simulink model "sampleModel7293_pp_1_1_mu"  (R2018a)
settings: Solver=VariableStepAuto  StartTime=0.0  StopTime=10.0  RelTol=1e-3
undefined symbols (not defined in the file): DiscIntNeverNeededParam
libraries: simulink x367
(part 3 of 13)

== system sampleModel7293_pp_1_1_mu/cfblk181 ==
  cfblk1 : Inport
  Action Port : ActionPort  ActionType=else
  cfblk10 : Subsystem  TreatAsAtomicUnit=on
  cfblk3 : simulink/Continuous/PID Controller (2DOF)  Controller=PID  TimeDomain=Discrete-time  SampleTime=-1  IntegratorMethod=Forward Euler  FilterMethod=Forward Euler  Form=Parallel  UseFilter=on  ControllerParametersSource=internal  P=1  I=1  D=0  N=100  b=1  c=1  InitialConditionSource=internal  InitialConditionForIntegrator=0  InitialConditionForFilter=0  ExternalReset=none  LimitOutput=off  UpperSaturationLimit=inf  LowerSaturationLimit=-inf  LinearizeAsGain=off  AntiWindupMode=none  Kb=1  TrackingMode=off  Kt=1  PParamMin=[]  PParamMax=[]  IParamMin=[]  IParamMax=[]  DParamMin=[]  DParamMax=[]  NParamMin=[]  NParamMax=[]  bParamMin=[]  bParamMax=[]  cParamMin=[]  cParamMax=[]  KbParamMin=[]  KbParamMax=[]  KtParamMin=[]  KtParamMax=[]  POutMin=[]  POutMax=[]  IOutMin=[]  IOutMax=[]  DOutMin=[]  DOutMax=[]  NOutMin=[]  NOutMax=[]  bOutMin=[]  bOutMax=[]  cOutMin=[]  cOutMax=[]  KbOutMin=[]  KbOutMax=[]  KtOutMin=[]  KtOutMax=[]  IntegratorOutMin=[]  IntegratorOutMax=[]  FilterOutMin=[]  FilterOutMax=[]  SumOutMin=[]  SumOutMax=[]  Sum1OutMin=[]  Sum1OutMax=[]  Sum2OutMin=[]  Sum2OutMax=[]  Sum3OutMin=[]  Sum3OutMax=[]  SumI1OutMin=[]  SumI1OutMax=[]  SumI2OutMin=[]  SumI2OutMax=[]  SumI3OutMin=[]  SumI3OutMax=[]  SumDOutMin=[]  SumDOutMax=[]  SaturationOutMin=[]  SaturationOutMax=[]  IntegratorContinuousStateAttributes=''  IntegratorStateMustResolveToSignalObject=off  IntegratorRTWStateStorageClass=Auto  FilterContinuousStateAttributes=''  FilterStateMustResolveToSignalObject=off  FilterRTWStateStorageClass=Auto  DifferentiatorICPrevScaledInput=0  DifferentiatorOutMin=[]  DifferentiatorOutMax=[]  FilterDiffOutCoefMin=[]  FilterDiffOutCoefMax=[]  SumDenOutMin=[]  SumDenOutMax=[]  SumNumOutMin=[]  SumNumOutMax=[]  ReciprocalOutMin=[]  ReciprocalOutMax=[]  DivideOutMin=[]  DivideOutMax=[]  TunerSelectOption=Transfer Function Based (PID Tuner App)
  cfblk4 : DiscreteFilter
  cfblk5 : Delay  DelayLengthSource=Input port
      settings: InputPortMap=u0,p1
  cfblk6 : DiscreteFilter
  cfblk7 : Delay  ShowEnablePort=on
      settings: InputPortMap=u0,e6
  cfblk8 : DiscreteTransferFcn
  cyemi_{464..473} (10 alike) : DataTypeConversion  OutDataTypeStr=double
  emi_81 : Subsystem  TreatAsAtomicUnit=on
  emi_83 : If  IfExpression=0 <= u1
  emi_84 : DataTypeConversion  OutDataTypeStr=double
  cfblk2 : Outport
  cfblk9 : Outport  Port=2
  wires:
  cfblk4/1 -> cfblk9/1
  cfblk1/1 -> cyemi_466/1, cyemi_468/1
  cfblk5/1 -> cyemi_470/1, cyemi_472/1
  cfblk3/1 -> cfblk2/1, cyemi_471/1
  cfblk7/1 -> cyemi_464/1, cyemi_467/1
  cyemi_465/1 -> cfblk3/1
  cfblk8/1 -> cyemi_465/1
  cyemi_466/1 -> cfblk3/2
  cyemi_467/1 -> cfblk4/1
  cyemi_468/1 -> cfblk5/1
  cyemi_469/1 -> cfblk5/2
  cyemi_470/1 -> cfblk6/1
  cyemi_471/1 -> cfblk7/1
  cyemi_472/1 -> cfblk7/2
  cyemi_473/1 -> cfblk8/1
  cfblk6/1 -> cyemi_473/1, emi_84/1
  cyemi_464/1 -> cfblk10/1(emi_79)
  cfblk10/1(emi_80) -> cyemi_469/1
  emi_83/1 -> cfblk10/Action
  emi_83/2 -> emi_81/Action
  emi_84/1 -> emi_83/1

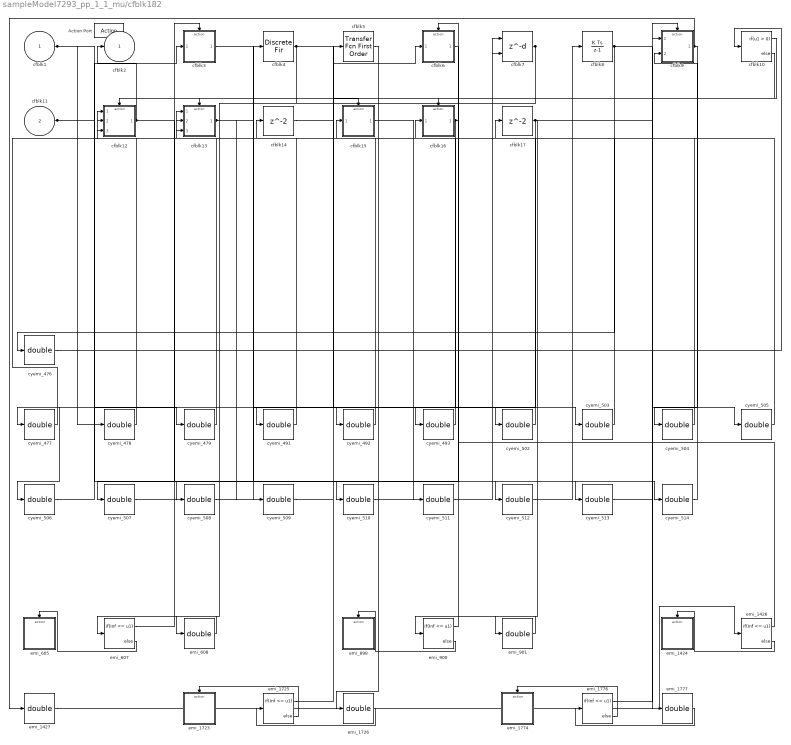
== system sampleModel7293_pp_1_1_mu/cfblk182 ==
  cfblk1 : Inport
  cfblk11 : Inport  Port=2
  Action Port : ActionPort  ActionType=then
  cfblk10 : If  SampleTime=1
  cfblk12 : Subsystem  TreatAsAtomicUnit=on
  cfblk13 : Subsystem  TreatAsAtomicUnit=on
  cfblk14 : Delay
  cfblk15 : Subsystem  TreatAsAtomicUnit=on
  cfblk16 : Subsystem  TreatAsAtomicUnit=on
  cfblk17 : Delay
  cfblk3 : Subsystem  TreatAsAtomicUnit=on
  cfblk4 : DiscreteFir
  cfblk5 : simulink/Discrete/Transfer Fcn First Order  PoleZ=0.95  ICPrevOutput=0.0  DoSatur=off
      settings: SourceProductName=Simulink
  cfblk6 : Subsystem  TreatAsAtomicUnit=on
  cfblk7 : Delay  DelayLengthSource=Input port
      settings: InputPortMap=u0,p1
  cfblk8 : DiscreteIntegrator  SampleTime=-1  OutDataTypeStr=double  ICPrevOutput=DiscIntNeverNeededParam  ICPrevScaledInput=DiscIntNeverNeededParam
  cfblk9 : Subsystem  TreatAsAtomicUnit=on
  cyemi_{476..479,491..493,502..514} (20 alike) : DataTypeConversion  OutDataTypeStr=double
  emi_1424 : Subsystem  TreatAsAtomicUnit=on
  emi_{607,900,1426,1725,1776} (5 alike) : If  IfExpression=Inf <= u1
  emi_{608,901,1427,1726,1777} (5 alike) : DataTypeConversion  OutDataTypeStr=double
  emi_1723 : Subsystem  TreatAsAtomicUnit=on
  emi_1774 : Subsystem  TreatAsAtomicUnit=on
  emi_605 : Subsystem  TreatAsAtomicUnit=on
  emi_898 : Subsystem  TreatAsAtomicUnit=on
  cfblk2 : Outport
  wires:
  cfblk13/1(cfblk2) -> cyemi_503/1, cyemi_509/1
  cfblk1/1 -> cyemi_478/1, cyemi_510/1
  cfblk12/1(cfblk2) -> cfblk2/1, cyemi_514/1
  cfblk8/1 -> cyemi_476/1, cyemi_505/1
  cfblk11/1 -> cyemi_479/1, cyemi_513/1
  cfblk7/1 -> cyemi_477/1, cyemi_508/1
  cfblk10/1 -> cfblk12/Action
  cfblk10/2 -> cfblk13/Action
  cyemi_476/1 -> cfblk10/1
  cyemi_477/1 -> cfblk12/1(cfblk1)
  cyemi_478/1 -> cfblk12/2(cfblk13)
  cyemi_479/1 -> cfblk12/3(cfblk14)
  cyemi_491/1 -> cfblk13/1(cfblk1)
  cyemi_492/1 -> cfblk13/2(cfblk9)
  cfblk5/1 -> cyemi_492/1
  cyemi_493/1 -> cfblk13/3(cfblk10)
  cfblk14/1 -> cyemi_493/1
  cyemi_502/1 -> cfblk14/1
  cfblk4/1 -> cyemi_502/1, emi_608/1
  cyemi_505/1 -> cfblk17/1
  cfblk17/1 -> cyemi_506/1, emi_901/1, emi_1777/1
  cyemi_507/1 -> cfblk4/1
  cyemi_508/1 -> cfblk5/1
  cyemi_510/1 -> cfblk7/1
  cyemi_511/1 -> cfblk7/2
  cyemi_512/1 -> cfblk8/1
  cyemi_506/1 -> cfblk3/1(emi_603)
  cfblk3/1(emi_604) -> cyemi_512/1
  emi_607/1 -> cfblk3/Action
  emi_607/2 -> emi_605/Action
  emi_608/1 -> emi_607/1
  cyemi_509/1 -> cfblk6/1(emi_896)
  cfblk6/1(emi_897) -> cyemi_507/1
  emi_900/1 -> cfblk6/Action
  emi_900/2 -> emi_898/Action
  emi_901/1 -> emi_900/1
  cyemi_504/1 -> cfblk16/1(emi_1422)
  cfblk16/1(emi_1423) -> cyemi_491/1, emi_1726/1
  emi_1426/1 -> cfblk16/Action
  emi_1426/2 -> emi_1424/Action
  emi_1427/1 -> emi_1426/1
  cyemi_503/1 -> cfblk15/1(emi_1721)
  cfblk15/1(emi_1722) -> cyemi_511/1
  emi_1725/1 -> cfblk15/Action
  emi_1725/2 -> emi_1723/Action
  emi_1726/1 -> emi_1725/1
  cyemi_513/1 -> cfblk9/1(emi_1771)
  cyemi_514/1 -> cfblk9/2(emi_1772)
  cfblk9/1(emi_1773) -> emi_1427/1, cyemi_504/1
  emi_1776/1 -> cfblk9/Action
  emi_1776/2 -> emi_1774/Action
  emi_1777/1 -> emi_1776/1

== system sampleModel7293_pp_1_1_mu/cfblk183 ==
  cfblk1 : Inport
  cfblk10 : Inport  Port=2
  cfblk11 : Inport  Port=3
  Action Port : ActionPort  ActionType=else
  cfblk15 : Subsystem  TreatAsAtomicUnit=on
  cfblk3 : Subsystem  TreatAsAtomicUnit=on
  cfblk4 : Subsystem  TreatAsAtomicUnit=on
  cfblk5 : Subsystem  TreatAsAtomicUnit=on
  cfblk6 : DiscreteStateSpace  SampleTime=-1
  cfblk7 : Delay
  cfblk8 : DiscreteStateSpace  SampleTime=-1
  cfblk9 : simulink/Continuous/PID Controller  Controller=PID  TimeDomain=Discrete-time  SampleTime=-1  IntegratorMethod=Forward Euler  FilterMethod=Forward Euler  Form=Parallel  UseFilter=on  ControllerParametersSource=internal  P=1  I=1  D=0  N=100  InitialConditionSource=internal  InitialConditionForIntegrator=0  InitialConditionForFilter=0  ExternalReset=none  LimitOutput=off  UpperSaturationLimit=inf  LowerSaturationLimit=-inf  LinearizeAsGain=off  AntiWindupMode=none  Kb=1  TrackingMode=off  Kt=1  PParamMin=[]  PParamMax=[]  IParamMin=[]  IParamMax=[]  DParamMin=[]  DParamMax=[]  NParamMin=[]  NParamMax=[]  KbParamMin=[]  KbParamMax=[]  KtParamMin=[]  KtParamMax=[]  POutMin=[]  POutMax=[]  IOutMin=[]  IOutMax=[]  DOutMin=[]  DOutMax=[]  NOutMin=[]  NOutMax=[]  KbOutMin=[]  KbOutMax=[]  KtOutMin=[]  KtOutMax=[]  IntegratorOutMin=[]  IntegratorOutMax=[]  FilterOutMin=[]  FilterOutMax=[]  SumOutMin=[]  SumOutMax=[]  SumI1OutMin=[]  SumI1OutMax=[]  SumI2OutMin=[]  SumI2OutMax=[]  SumI3OutMin=[]  SumI3OutMax=[]  SumDOutMin=[]  SumDOutMax=[]  SaturationOutMin=[]  SaturationOutMax=[]  IntegratorContinuousStateAttributes=''  IntegratorStateMustResolveToSignalObject=off  IntegratorRTWStateStorageClass=Auto  FilterContinuousStateAttributes=''  FilterStateMustResolveToSignalObject=off  FilterRTWStateStorageClass=Auto  DifferentiatorICPrevScaledInput=0  DifferentiatorOutMin=[]  DifferentiatorOutMax=[]  FilterDiffOutCoefMin=[]  FilterDiffOutCoefMax=[]  SumDenOutMin=[]  SumDenOutMax=[]  SumNumOutMin=[]  SumNumOutMax=[]  ReciprocalOutMin=[]  ReciprocalOutMax=[]  DivideOutMin=[]  DivideOutMax=[]  TunerSelectOption=Transfer Function Based (PID Tuner App)
  cyemi_{518..526} (9 alike) : DataTypeConversion  OutDataTypeStr=double
  emi_1403 : Subsystem  TreatAsAtomicUnit=on
  emi_{398,1405,1854,1966} (4 alike) : If  IfExpression=0 <= u1
  emi_{399,1406,1855,1967} (4 alike) : DataTypeConversion  OutDataTypeStr=double
  emi_1852 : Subsystem  TreatAsAtomicUnit=on
  emi_1964 : Subsystem  TreatAsAtomicUnit=on
  emi_396 : Subsystem  TreatAsAtomicUnit=on
  cfblk2 : Outport
  cfblk12 : Outport  Port=2
  cfblk13 : Outport  Port=3
  cfblk14 : Outport  Port=4
  wires:
  cfblk1/1 -> cfblk14/1
  cfblk7/1 -> cfblk2/1, cyemi_525/1
  cfblk8/1 -> cyemi_518/1
  cfblk10/1 -> cyemi_520/1
  cfblk6/1 -> cyemi_521/1
  cfblk9/1 -> cyemi_522/1
  cyemi_523/1 -> cfblk6/1
  cfblk11/1 -> cyemi_523/1
  cyemi_524/1 -> cfblk7/1
  cyemi_525/1 -> cfblk8/1
  cyemi_526/1 -> cfblk9/1
  cyemi_521/1 -> cfblk4/1(emi_394)
  cfblk4/1(emi_395) -> cfblk12/1
  emi_398/1 -> cfblk4/Action
  emi_398/2 -> emi_396/Action
  emi_399/1 -> emi_398/1
  cyemi_519/1 -> cfblk3/1(emi_1400)
  cyemi_520/1 -> cfblk3/2(emi_1401)
  cfblk3/1(emi_1402) -> cyemi_526/1, emi_1967/1
  emi_1405/1 -> cfblk3/Action
  emi_1405/2 -> emi_1403/Action
  emi_1406/1 -> emi_1405/1
  cyemi_518/1 -> cfblk15/1(emi_1850)
  cfblk15/1(emi_1851) -> emi_1406/1, emi_399/1, cyemi_519/1
  emi_1854/1 -> cfblk15/Action
  emi_1854/2 -> emi_1852/Action
  emi_1855/1 -> emi_1854/1
  cyemi_522/1 -> cfblk5/1(emi_1962)
  cfblk5/1(emi_1963) -> emi_1855/1, cyemi_524/1, cfblk13/1
  emi_1966/1 -> cfblk5/Action
  emi_1966/2 -> emi_1964/Action
  emi_1967/1 -> emi_1966/1

== system sampleModel7293_pp_1_1_mu/cfblk184 ==
  cfblk1 : Inport
  Action Port : ActionPort  ActionType=then
  cfblk10 : UnitDelay  SampleTime=-1
  cfblk11 : Delay  DelayLengthSource=Input port
      settings: InputPortMap=u0,p1
  cfblk12 : Subsystem  TreatAsAtomicUnit=on
  cfblk13 : DiscreteStateSpace  SampleTime=-1
  cfblk14 : simulink/Discrete/Transfer Fcn First Order  PoleZ=0.95  ICPrevOutput=0.0  DoSatur=off
      settings: SourceProductName=Simulink
  cfblk15 : If  SampleTime=1
  cfblk16 : Subsystem  TreatAsAtomicUnit=on
  cfblk17 : Subsystem  TreatAsAtomicUnit=on
  cfblk{18..22} (5 alike) : Delay
  cfblk3 : DiscreteIntegrator  SampleTime=-1  OutDataTypeStr=double  ICPrevOutput=DiscIntNeverNeededParam  ICPrevScaledInput=DiscIntNeverNeededParam
  cfblk4 : Delay  DelayLengthSource=Input port
      settings: InputPortMap=u0,p1
  cfblk5 : simulink/Discrete/Difference  ICPrevInput=0.0  OutMin=[]  OutMax=[]  OutDataTypeStr=double  OutputDataTypeScalingMode=double  OutDataType=fixdt(1, 16)  OutScaling=2^-10  DoSatur=off
  cfblk6 : simulink/Discrete/Transfer Fcn Lead or Lag  PoleZ=0.95  ZeroZ=0.75  ICPrevOutput=0.0  ICPrevInput=0.0  DoSatur=off
      settings: SourceProductName=Simulink  SourceProductBaseCode=SL
  cfblk7 : simulink/Discrete/Transfer Fcn Real Zero  ZeroZ=0.75  ICPrevInput=0.0  DoSatur=off
      settings: SourceProductName=Simulink  SourceProductBaseCode=SL
  cfblk8 : Subsystem  TreatAsAtomicUnit=on
  cfblk9 : simulink/Discrete/Transfer Fcn Lead or Lag  PoleZ=0.95  ZeroZ=0.75  ICPrevOutput=0.0  ICPrevInput=0.0  DoSatur=off
      settings: SourceProductName=Simulink  SourceProductBaseCode=SL
  cyemi_{528..536,555,572..584} (23 alike) : DataTypeConversion  OutDataTypeStr=double
  emi_1751 : Subsystem  TreatAsAtomicUnit=on
  emi_1753 : If  IfExpression=Inf <= u1
  emi_1754 : DataTypeConversion  OutDataTypeStr=double
  emi_856 : Subsystem  TreatAsAtomicUnit=on
  emi_858 : If  IfExpression=Inf <= u1
  emi_859 : DataTypeConversion  OutDataTypeStr=double
  cfblk2 : Outport
  wires:
  cfblk14/1 -> cyemi_531/1, cyemi_573/1
  cfblk9/1 -> cyemi_532/1, cyemi_576/1
  cfblk10/1 -> cfblk2/1
  cfblk15/1 -> cfblk16/Action
  cfblk15/2 -> cfblk17/Action
  cyemi_528/1 -> cfblk10/1
  cfblk16/1(cfblk2) -> cyemi_528/1
  cyemi_529/1 -> cfblk11/1
  cfblk19/1 -> cyemi_529/1
  cyemi_530/1 -> cfblk11/2
  cfblk1/1 -> cyemi_530/1
  cyemi_533/1 -> cfblk13/1
  cfblk5/1 -> cyemi_533/1
  cyemi_534/1 -> cfblk14/1
  cfblk13/1 -> cyemi_534/1
  cyemi_535/1 -> cfblk15/1
  cfblk18/1 -> cyemi_535/1
  cyemi_536/1 -> cfblk16/1(cfblk1)
  cfblk4/1 -> cyemi_536/1
  cyemi_555/1 -> cfblk17/1(cfblk1)
  cfblk21/1 -> cyemi_555/1
  cyemi_572/1 -> cfblk18/1
  cfblk16/2(cfblk16) -> cyemi_572/1
  cyemi_573/1 -> cfblk19/1
  cyemi_574/1 -> cfblk20/1
  cyemi_575/1 -> cfblk21/1
  cyemi_576/1 -> cfblk22/1
  cyemi_577/1 -> cfblk3/1
  cfblk6/1 -> cyemi_577/1
  cyemi_578/1 -> cfblk4/1
  cfblk20/1 -> cyemi_578/1
  cyemi_579/1 -> cfblk4/2
  cfblk11/1 -> cyemi_579/1, emi_1754/1
  cyemi_580/1 -> cfblk5/1
  cfblk3/1 -> cyemi_580/1
  cyemi_581/1 -> cfblk6/1
  cfblk17/1(cfblk2) -> cyemi_581/1
  cyemi_582/1 -> cfblk7/1
  cfblk22/1 -> cyemi_582/1
  cfblk17/2(cfblk15) -> cyemi_583/1
  cyemi_584/1 -> cfblk9/1
  cfblk7/1 -> cyemi_584/1
  cyemi_531/1 -> cfblk12/1(emi_853)
  cyemi_532/1 -> cfblk12/2(emi_854)
  cfblk12/1(emi_855) -> cyemi_574/1
  emi_858/1 -> cfblk12/Action
  emi_858/2 -> emi_856/Action
  emi_859/1 -> emi_858/1
  cyemi_583/1 -> cfblk8/1(emi_1749)
  cfblk8/1(emi_1750) -> emi_859/1, cyemi_575/1
  emi_1753/1 -> cfblk8/Action
  emi_1753/2 -> emi_1751/Action
  emi_1754/1 -> emi_1753/1

== system sampleModel7293_pp_1_1_mu/cfblk185 ==
  cfblk1 : Inport
  cfblk12 : Inport  Port=2
  cfblk13 : Inport  Port=3
  cfblk14 : Inport  Port=4
  cfblk15 : Inport  Port=5
  cfblk16 : Inport  Port=6
  Action Port : ActionPort  ActionType=else
  cfblk10 : Delay  DelayLengthSource=Input port
      settings: InputPortMap=u0,p1
  cfblk11 : If  SampleTime=1
  cfblk18 : Subsystem  TreatAsAtomicUnit=on
  cfblk19 : Subsystem  TreatAsAtomicUnit=on
  cfblk20 : Delay
  cfblk3 : simulink/Discrete/Transfer Fcn First Order  PoleZ=0.95  ICPrevOutput=0.0  DoSatur=off
      settings: SourceProductName=Simulink
  cfblk4 : simulink/Continuous/PID Controller (2DOF)  Controller=PID  TimeDomain=Discrete-time  SampleTime=-1  IntegratorMethod=Forward Euler  FilterMethod=Forward Euler  Form=Parallel  UseFilter=on  ControllerParametersSource=internal  P=1  I=1  D=0  N=100  b=1  c=1  InitialConditionSource=internal  InitialConditionForIntegrator=0  InitialConditionForFilter=0  ExternalReset=none  LimitOutput=off  UpperSaturationLimit=inf  LowerSaturationLimit=-inf  LinearizeAsGain=off  AntiWindupMode=none  Kb=1  TrackingMode=off  Kt=1  PParamMin=[]  PParamMax=[]  IParamMin=[]  IParamMax=[]  DParamMin=[]  DParamMax=[]  NParamMin=[]  NParamMax=[]  bParamMin=[]  bParamMax=[]  cParamMin=[]  cParamMax=[]  KbParamMin=[]  KbParamMax=[]  KtParamMin=[]  KtParamMax=[]  POutMin=[]  POutMax=[]  IOutMin=[]  IOutMax=[]  DOutMin=[]  DOutMax=[]  NOutMin=[]  NOutMax=[]  bOutMin=[]  bOutMax=[]  cOutMin=[]  cOutMax=[]  KbOutMin=[]  KbOutMax=[]  KtOutMin=[]  KtOutMax=[]  IntegratorOutMin=[]  IntegratorOutMax=[]  FilterOutMin=[]  FilterOutMax=[]  SumOutMin=[]  SumOutMax=[]  Sum1OutMin=[]  Sum1OutMax=[]  Sum2OutMin=[]  Sum2OutMax=[]  Sum3OutMin=[]  Sum3OutMax=[]  SumI1OutMin=[]  SumI1OutMax=[]  SumI2OutMin=[]  SumI2OutMax=[]  SumI3OutMin=[]  SumI3OutMax=[]  SumDOutMin=[]  SumDOutMax=[]  SaturationOutMin=[]  SaturationOutMax=[]  IntegratorContinuousStateAttributes=''  IntegratorStateMustResolveToSignalObject=off  IntegratorRTWStateStorageClass=Auto  FilterContinuousStateAttributes=''  FilterStateMustResolveToSignalObject=off  FilterRTWStateStorageClass=Auto  DifferentiatorICPrevScaledInput=0  DifferentiatorOutMin=[]  DifferentiatorOutMax=[]  FilterDiffOutCoefMin=[]  FilterDiffOutCoefMax=[]  SumDenOutMin=[]  SumDenOutMax=[]  SumNumOutMin=[]  SumNumOutMax=[]  ReciprocalOutMin=[]  ReciprocalOutMax=[]  DivideOutMin=[]  DivideOutMax=[]  TunerSelectOption=Transfer Function Based (PID Tuner App)
  cfblk5 : simulink/Discrete/Tapped Delay  vinit=0.0  samptime=-1  NumDelays=1  DelayOrder=Oldest  includeCurrent=off
  cfblk6 : simulink/Discrete/Transfer Fcn Lead or Lag  PoleZ=0.95  ZeroZ=0.75  ICPrevOutput=0.0  ICPrevInput=0.0  DoSatur=off
      settings: SourceProductName=Simulink  SourceProductBaseCode=SL
  cfblk7 : simulink/Continuous/PID Controller (2DOF)  Controller=PID  TimeDomain=Discrete-time  SampleTime=-1  IntegratorMethod=Forward Euler  FilterMethod=Forward Euler  Form=Parallel  UseFilter=on  ControllerParametersSource=internal  P=1  I=1  D=0  N=100  b=1  c=1  InitialConditionSource=internal  InitialConditionForIntegrator=0  InitialConditionForFilter=0  ExternalReset=none  LimitOutput=off  UpperSaturationLimit=inf  LowerSaturationLimit=-inf  LinearizeAsGain=off  AntiWindupMode=none  Kb=1  TrackingMode=off  Kt=1  PParamMin=[]  PParamMax=[]  IParamMin=[]  IParamMax=[]  DParamMin=[]  DParamMax=[]  NParamMin=[]  NParamMax=[]  bParamMin=[]  bParamMax=[]  cParamMin=[]  cParamMax=[]  KbParamMin=[]  KbParamMax=[]  KtParamMin=[]  KtParamMax=[]  POutMin=[]  POutMax=[]  IOutMin=[]  IOutMax=[]  DOutMin=[]  DOutMax=[]  NOutMin=[]  NOutMax=[]  bOutMin=[]  bOutMax=[]  cOutMin=[]  cOutMax=[]  KbOutMin=[]  KbOutMax=[]  KtOutMin=[]  KtOutMax=[]  IntegratorOutMin=[]  IntegratorOutMax=[]  FilterOutMin=[]  FilterOutMax=[]  SumOutMin=[]  SumOutMax=[]  Sum1OutMin=[]  Sum1OutMax=[]  Sum2OutMin=[]  Sum2OutMax=[]  Sum3OutMin=[]  Sum3OutMax=[]  SumI1OutMin=[]  SumI1OutMax=[]  SumI2OutMin=[]  SumI2OutMax=[]  SumI3OutMin=[]  SumI3OutMax=[]  SumDOutMin=[]  SumDOutMax=[]  SaturationOutMin=[]  SaturationOutMax=[]  IntegratorContinuousStateAttributes=''  IntegratorStateMustResolveToSignalObject=off  IntegratorRTWStateStorageClass=Auto  FilterContinuousStateAttributes=''  FilterStateMustResolveToSignalObject=off  FilterRTWStateStorageClass=Auto  DifferentiatorICPrevScaledInput=0  DifferentiatorOutMin=[]  DifferentiatorOutMax=[]  FilterDiffOutCoefMin=[]  FilterDiffOutCoefMax=[]  SumDenOutMin=[]  SumDenOutMax=[]  SumNumOutMin=[]  SumNumOutMax=[]  ReciprocalOutMin=[]  ReciprocalOutMax=[]  DivideOutMin=[]  DivideOutMax=[]  TunerSelectOption=Transfer Function Based (PID Tuner App)
  cfblk8 : DiscreteFilter
  cfblk9 : DiscreteTransferFcn
  cyemi_{591..595,607,616..625} (16 alike) : DataTypeConversion  OutDataTypeStr=double
  cfblk2 : Outport
  cfblk17 : Outport  Port=2
  wires:
  cfblk7/1 -> cfblk17/1
  cfblk6/1 -> cfblk2/1
  cfblk11/1 -> cfblk18/Action
  cfblk11/2 -> cfblk19/Action
  cyemi_591/1 -> cfblk10/1
  cfblk19/1(cfblk2) -> cyemi_591/1
  cyemi_592/1 -> cfblk10/2
  cfblk4/1 -> cyemi_592/1
  cyemi_593/1 -> cfblk11/1
  cfblk5/1 -> cyemi_593/1
  cyemi_594/1 -> cfblk18/1(cfblk1)
  cfblk9/1 -> cyemi_594/1
  cyemi_595/1 -> cfblk18/2(cfblk11)
  cfblk12/1 -> cyemi_595/1
  cyemi_607/1 -> cfblk19/1(cfblk1)
  cfblk18/2(cfblk12) -> cyemi_607/1
  cyemi_616/1 -> cfblk20/1
  cfblk18/1(cfblk2) -> cyemi_616/1
  cyemi_617/1 -> cfblk3/1
  cfblk20/1 -> cyemi_617/1
  cyemi_618/1 -> cfblk4/1
  cfblk16/1 -> cyemi_618/1
  cyemi_619/1 -> cfblk4/2
  cfblk13/1 -> cyemi_619/1
  cyemi_620/1 -> cfblk5/1
  cfblk8/1 -> cyemi_620/1
  cyemi_621/1 -> cfblk6/1
  cfblk15/1 -> cyemi_621/1
  cyemi_622/1 -> cfblk7/1
  cfblk1/1 -> cyemi_622/1
  cyemi_623/1 -> cfblk7/2
  cfblk10/1 -> cyemi_623/1
  cyemi_624/1 -> cfblk8/1
  cfblk14/1 -> cyemi_624/1
  cyemi_625/1 -> cfblk9/1
  cfblk3/1 -> cyemi_625/1

== system sampleModel7293_pp_1_1_mu/cfblk186 ==
  cfblk1 : Inport
  cfblk5 : Inport  Port=2
  cfblk6 : Inport  Port=3
  cfblk7 : Inport  Port=4
  Action Port : ActionPort  ActionType=then
  cfblk3 : Delay  ShowEnablePort=on
      settings: InputPortMap=u0,e6
  cfblk4 : simulink/Discrete/Difference  ICPrevInput=0.0  OutMin=[]  OutMax=[]  OutDataTypeStr=double  OutputDataTypeScalingMode=double  OutDataType=fixdt(1, 16)  OutScaling=2^-10  DoSatur=off
  cyemi_630 : DataTypeConversion  OutDataTypeStr=double
  cyemi_631 : DataTypeConversion  OutDataTypeStr=double
  cyemi_632 : DataTypeConversion  OutDataTypeStr=double
  cfblk2 : Outport
  cfblk8 : Outport  Port=2
  wires:
  cfblk5/1 -> cfblk2/1
  cfblk7/1 -> cfblk8/1
  cyemi_630/1 -> cfblk3/1
  cfblk1/1 -> cyemi_630/1
  cyemi_631/1 -> cfblk3/2
  cfblk4/1 -> cyemi_631/1
  cyemi_632/1 -> cfblk4/1
  cfblk6/1 -> cyemi_632/1

== system sampleModel7293_pp_1_1_mu/cfblk187 ==
  cfblk1 : Inport
  cfblk8 : Inport  Port=2
  cfblk9 : Inport  Port=3
  Action Port : ActionPort  ActionType=else
  cfblk11 : Subsystem  TreatAsAtomicUnit=on
  cfblk12 : Subsystem  TreatAsAtomicUnit=on
  cfblk13 : Delay
  cfblk14 : Subsystem  TreatAsAtomicUnit=on
  cfblk15 : Delay
  cfblk3 : Subsystem  TreatAsAtomicUnit=on
  cfblk4 : simulink/Discrete/Tapped Delay  vinit=0.0  samptime=-1  NumDelays=1  DelayOrder=Oldest  includeCurrent=off
  cfblk5 : simulink/Continuous/PID Controller (2DOF)  Controller=PID  TimeDomain=Discrete-time  SampleTime=-1  IntegratorMethod=Forward Euler  FilterMethod=Forward Euler  Form=Parallel  UseFilter=on  ControllerParametersSource=internal  P=1  I=1  D=0  N=100  b=1  c=1  InitialConditionSource=internal  InitialConditionForIntegrator=0  InitialConditionForFilter=0  ExternalReset=none  LimitOutput=off  UpperSaturationLimit=inf  LowerSaturationLimit=-inf  LinearizeAsGain=off  AntiWindupMode=none  Kb=1  TrackingMode=off  Kt=1  PParamMin=[]  PParamMax=[]  IParamMin=[]  IParamMax=[]  DParamMin=[]  DParamMax=[]  NParamMin=[]  NParamMax=[]  bParamMin=[]  bParamMax=[]  cParamMin=[]  cParamMax=[]  KbParamMin=[]  KbParamMax=[]  KtParamMin=[]  KtParamMax=[]  POutMin=[]  POutMax=[]  IOutMin=[]  IOutMax=[]  DOutMin=[]  DOutMax=[]  NOutMin=[]  NOutMax=[]  bOutMin=[]  bOutMax=[]  cOutMin=[]  cOutMax=[]  KbOutMin=[]  KbOutMax=[]  KtOutMin=[]  KtOutMax=[]  IntegratorOutMin=[]  IntegratorOutMax=[]  FilterOutMin=[]  FilterOutMax=[]  SumOutMin=[]  SumOutMax=[]  Sum1OutMin=[]  Sum1OutMax=[]  Sum2OutMin=[]  Sum2OutMax=[]  Sum3OutMin=[]  Sum3OutMax=[]  SumI1OutMin=[]  SumI1OutMax=[]  SumI2OutMin=[]  SumI2OutMax=[]  SumI3OutMin=[]  SumI3OutMax=[]  SumDOutMin=[]  SumDOutMax=[]  SaturationOutMin=[]  SaturationOutMax=[]  IntegratorContinuousStateAttributes=''  IntegratorStateMustResolveToSignalObject=off  IntegratorRTWStateStorageClass=Auto  FilterContinuousStateAttributes=''  FilterStateMustResolveToSignalObject=off  FilterRTWStateStorageClass=Auto  DifferentiatorICPrevScaledInput=0  DifferentiatorOutMin=[]  DifferentiatorOutMax=[]  FilterDiffOutCoefMin=[]  FilterDiffOutCoefMax=[]  SumDenOutMin=[]  SumDenOutMax=[]  SumNumOutMin=[]  SumNumOutMax=[]  ReciprocalOutMin=[]  ReciprocalOutMax=[]  DivideOutMin=[]  DivideOutMax=[]  TunerSelectOption=Transfer Function Based (PID Tuner App)
  cfblk6 : DiscreteFilter
  cfblk7 : If  SampleTime=1
  cyemi_{636..638,651..653,660..669} (16 alike) : DataTypeConversion  OutDataTypeStr=double
  emi_339 : Subsystem  TreatAsAtomicUnit=on
  emi_341 : If  IfExpression=0 <= u1
  emi_342 : DataTypeConversion  OutDataTypeStr=double
  emi_776 : Subsystem  TreatAsAtomicUnit=on
  emi_778 : If  IfExpression=0 <= u1
  emi_779 : DataTypeConversion  OutDataTypeStr=double
  cfblk2 : Outport
  cfblk10 : Outport  Port=2
  wires:
  cfblk9/1 -> cyemi_638/1, cyemi_669/1
  cfblk6/1 -> cfblk2/1, cyemi_637/1, cyemi_666/1, emi_342/1
  cfblk12/2(cfblk10) -> cyemi_660/1, cyemi_664/1
  cfblk4/1 -> cyemi_661/1, cyemi_662/1, emi_779/1
  cfblk7/1 -> cfblk11/Action
  cfblk7/2 -> cfblk12/Action
  cyemi_636/1 -> cfblk11/1(cfblk1)
  cfblk8/1 -> cyemi_636/1
  cyemi_637/1 -> cfblk11/2(cfblk13)
  cyemi_638/1 -> cfblk11/3(cfblk14)
  cyemi_651/1 -> cfblk12/1(cfblk1)
  cfblk5/1 -> cyemi_651/1
  cyemi_652/1 -> cfblk12/2(cfblk8)
  cyemi_653/1 -> cfblk12/3(cfblk9)
  cfblk15/1 -> cyemi_653/1
  cyemi_660/1 -> cfblk13/1
  cyemi_662/1 -> cfblk15/1
  cfblk12/1(cfblk2) -> cyemi_663/1
  cyemi_665/1 -> cfblk4/1
  cfblk11/1(cfblk2) -> cyemi_665/1
  cyemi_666/1 -> cfblk5/1
  cyemi_667/1 -> cfblk5/2
  cfblk13/1 -> cyemi_667/1
  cyemi_668/1 -> cfblk6/1
  cfblk1/1 -> cyemi_668/1
  cyemi_669/1 -> cfblk7/1
  cyemi_663/1 -> cfblk3/1(emi_336)
  cyemi_664/1 -> cfblk3/2(emi_337)
  cfblk3/1(emi_338) -> cfblk10/1
  emi_341/1 -> cfblk3/Action
  emi_341/2 -> emi_339/Action
  emi_342/1 -> emi_341/1
  cyemi_661/1 -> cfblk14/1(emi_774)
  cfblk14/1(emi_775) -> cyemi_652/1
  emi_778/1 -> cfblk14/Action
  emi_778/2 -> emi_776/Action
  emi_779/1 -> emi_778/1

== system sampleModel7293_pp_1_1_mu/cfblk188 ==
  cfblk1 : Inport
  cfblk9 : Inport  Port=2
  cfblk10 : Inport  Port=3
  cfblk11 : Inport  Port=4
  Action Port : ActionPort  ActionType=then
  cfblk3 : Subsystem  TreatAsAtomicUnit=on
  cfblk4 : Subsystem  TreatAsAtomicUnit=on
  cfblk5 : Subsystem  TreatAsAtomicUnit=on
  cfblk6 : Subsystem  TreatAsAtomicUnit=on
  cfblk7 : UnitDelay  SampleTime=-1
  cfblk8 : DiscreteIntegrator  SampleTime=-1  OutDataTypeStr=double  ICPrevOutput=DiscIntNeverNeededParam  ICPrevScaledInput=DiscIntNeverNeededParam
  cyemi_{674..679} (6 alike) : DataTypeConversion  OutDataTypeStr=double
  emi_1473 : Subsystem  TreatAsAtomicUnit=on
  emi_{182,454,650,1475} (4 alike) : If  IfExpression=Inf <= u1
  emi_{183,455,651,1476} (4 alike) : DataTypeConversion  OutDataTypeStr=double
  emi_180 : Subsystem  TreatAsAtomicUnit=on
  emi_452 : Subsystem  TreatAsAtomicUnit=on
  emi_648 : Subsystem  TreatAsAtomicUnit=on
  cfblk2 : Outport
  cfblk12 : Outport  Port=2
  wires:
  cfblk7/1 -> cfblk12/1
  cfblk1/1 -> cyemi_674/1
  cfblk8/1 -> cyemi_677/1, emi_651/1
  cyemi_678/1 -> cfblk7/1
  cfblk11/1 -> cyemi_678/1
  cyemi_679/1 -> cfblk8/1
  cyemi_677/1 -> cfblk6/1(emi_178)
  cfblk6/1(emi_179) -> cyemi_676/1
  emi_182/1 -> cfblk6/Action
  emi_182/2 -> emi_180/Action
  emi_183/1 -> emi_182/1
  cyemi_676/1 -> cfblk5/1(emi_450)
  cfblk5/1(emi_451) -> cyemi_675/1, emi_1476/1
  emi_454/1 -> cfblk5/Action
  emi_454/2 -> emi_452/Action
  emi_455/1 -> emi_454/1
  cyemi_674/1 -> cfblk3/1(emi_646)
  cfblk3/1(emi_647) -> emi_455/1, cyemi_679/1
  emi_650/1 -> cfblk3/Action
  emi_650/2 -> emi_648/Action
  emi_651/1 -> emi_650/1
  cyemi_675/1 -> cfblk4/1(emi_1471)
  cfblk4/1(emi_1472) -> emi_183/1, cfblk2/1
  emi_1475/1 -> cfblk4/Action
  emi_1475/2 -> emi_1473/Action
  emi_1476/1 -> emi_1475/1

== system sampleModel7293_pp_1_1_mu/cfblk189 ==
  cfblk1 : Inport
  cfblk12 : Inport  Port=2
  cfblk13 : Inport  Port=3
  Action Port : ActionPort  ActionType=else
  cfblk10 : Delay  DelayLengthSource=Input port
      settings: InputPortMap=u0,p1
  cfblk11 : If  SampleTime=1
  cfblk16 : Subsystem  TreatAsAtomicUnit=on
  cfblk17 : Subsystem  TreatAsAtomicUnit=on
  cfblk18 : Delay
  cfblk19 : Delay
  cfblk20 : Delay
  cfblk3 : DiscreteIntegrator  SampleTime=-1  OutDataTypeStr=double  ICPrevOutput=DiscIntNeverNeededParam  ICPrevScaledInput=DiscIntNeverNeededParam
  cfblk4 : Subsystem  TreatAsAtomicUnit=on
  cfblk5 : Subsystem  TreatAsAtomicUnit=on
  cfblk6 : simulink/Discrete/Transfer Fcn Real Zero  ZeroZ=0.75  ICPrevInput=0.0  DoSatur=off
      settings: SourceProductName=Simulink  SourceProductBaseCode=SL
  cfblk7 : DiscreteTransferFcn
  cfblk8 : simulink/Discrete/Transfer Fcn Lead or Lag  PoleZ=0.95  ZeroZ=0.75  ICPrevOutput=0.0  ICPrevInput=0.0  DoSatur=off
      settings: SourceProductName=Simulink  SourceProductBaseCode=SL
  cfblk9 : DiscreteIntegrator  SampleTime=-1  OutDataTypeStr=double  ICPrevOutput=DiscIntNeverNeededParam  ICPrevScaledInput=DiscIntNeverNeededParam
  cyemi_{683,685..689,699..700,716,718..726} (18 alike) : DataTypeConversion  OutDataTypeStr=double
  cyemi_684 : DataTypeConversion  OutDataTypeStr=uint32
  cyemi_717 : DataTypeConversion  OutDataTypeStr=uint32
  emi_1240 : Subsystem  TreatAsAtomicUnit=on
  emi_1242 : If  IfExpression=0 <= u1
  emi_1243 : DataTypeConversion  OutDataTypeStr=double
  emi_1510 : Subsystem  TreatAsAtomicUnit=on
  emi_1512 : If  IfExpression=0 <= u1
  emi_1513 : DataTypeConversion  OutDataTypeStr=uint32
  cfblk2 : Outport
  cfblk14 : Outport  Port=2
  cfblk15 : Outport  Port=3
  wires:
  cfblk1/1 -> cyemi_683/1, cyemi_687/1
  cfblk12/1 -> cfblk14/1
  cfblk7/1 -> cyemi_688/1, cyemi_718/1, cyemi_721/1, cyemi_725/1
  cfblk3/1 -> cyemi_699/1, cyemi_700/1, cyemi_724/1, emi_1243/1
  cfblk8/1 -> cfblk15/1, cyemi_689/1
  cfblk13/1 -> cfblk2/1
  cfblk11/1 -> cfblk16/Action
  cfblk11/2 -> cfblk17/Action
  cyemi_683/1 -> cfblk10/1
  cyemi_684/1 -> cfblk10/2
  cfblk19/1 -> cyemi_684/1, emi_1513/1
  cyemi_685/1 -> cfblk11/1
  cfblk10/1 -> cyemi_685/1
  cyemi_686/1 -> cfblk16/1(cfblk1)
  cfblk18/1 -> cyemi_686/1
  cyemi_687/1 -> cfblk16/2(cfblk11)
  cyemi_688/1 -> cfblk16/3(cfblk12)
  cyemi_689/1 -> cfblk16/4(cfblk13)
  cyemi_699/1 -> cfblk17/1(cfblk1)
  cyemi_700/1 -> cfblk17/2(cfblk15)
  cyemi_716/1 -> cfblk18/1
  cyemi_717/1 -> cfblk19/1
  cfblk17/1(cfblk2) -> cyemi_717/1
  cyemi_718/1 -> cfblk20/1
  cyemi_719/1 -> cfblk3/1
  cfblk20/1 -> cyemi_719/1
  cfblk6/1 -> cyemi_720/1
  cyemi_723/1 -> cfblk6/1
  cfblk9/1 -> cyemi_723/1
  cyemi_724/1 -> cfblk7/1
  cyemi_725/1 -> cfblk8/1
  cyemi_726/1 -> cfblk9/1
  cfblk16/1(cfblk2) -> cyemi_726/1
  cyemi_720/1 -> cfblk4/1(emi_1237)
  cyemi_721/1 -> cfblk4/2(emi_1238)
  cfblk4/1(emi_1239) -> cyemi_722/1
  emi_1242/1 -> cfblk4/Action
  emi_1242/2 -> emi_1240/Action
  emi_1243/1 -> emi_1242/1
  cyemi_722/1 -> cfblk5/1(emi_1508)
  cfblk5/1(emi_1509) -> cyemi_716/1
  emi_1512/1 -> cfblk5/Action
  emi_1512/2 -> emi_1510/Action
  emi_1513/1 -> emi_1512/1

== system sampleModel7293_pp_1_1_mu/cfblk190 ==
  cfblk1 : Inport
  Action Port : ActionPort  ActionType=then
  cfblk10 : Subsystem  TreatAsAtomicUnit=on
  cfblk11 : Delay
  cfblk12 : Subsystem  TreatAsAtomicUnit=on
  cfblk13 : Subsystem  TreatAsAtomicUnit=on
  cfblk3 : Subsystem  TreatAsAtomicUnit=on
  cfblk4 : UnitDelay  SampleTime=-1
  cfblk5 : Subsystem  TreatAsAtomicUnit=on
  cfblk6 : If  SampleTime=1
  cfblk9 : Subsystem  TreatAsAtomicUnit=on
  cyemi_{729..730,749..756} (10 alike) : DataTypeConversion  OutDataTypeStr=double
  emi_1802 : Subsystem  TreatAsAtomicUnit=on
  emi_{921,1804,2030,2144} (4 alike) : If  IfExpression=Inf <= u1
  emi_{922,1805,2031,2145} (4 alike) : DataTypeConversion  OutDataTypeStr=double
  emi_2028 : Subsystem  TreatAsAtomicUnit=on
  emi_2142 : Subsystem  TreatAsAtomicUnit=on
  emi_919 : Subsystem  TreatAsAtomicUnit=on
  cfblk2 : Outport
  cfblk7 : Outport  Port=2
  cfblk8 : Outport  Port=3
  wires:
  cfblk9/1(cfblk2) -> cfblk2/1, cyemi_754/1
  cfblk10/2(cfblk15) -> cfblk7/1, cyemi_753/1
  cfblk4/1 -> cfblk8/1, cyemi_751/1
  cfblk6/1 -> cfblk9/Action
  cfblk6/2 -> cfblk10/Action
  cyemi_729/1 -> cfblk10/1(cfblk1)
  cfblk11/1 -> cyemi_729/1
  cyemi_730/1 -> cfblk10/2(cfblk14)
  cfblk1/1 -> cyemi_730/1
  cyemi_749/1 -> cfblk11/1
  cfblk10/1(cfblk2) -> cyemi_750/1
  cyemi_753/1 -> cfblk4/1
  cyemi_755/1 -> cfblk6/1
  cyemi_756/1 -> cfblk9/1(cfblk1)
  cyemi_754/1 -> cfblk5/1(emi_917)
  cfblk5/1(emi_918) -> cyemi_752/1
  emi_921/1 -> cfblk5/Action
  emi_921/2 -> emi_919/Action
  emi_922/1 -> emi_921/1
  cyemi_751/1 -> cfblk13/1(emi_1800)
  cfblk13/1(emi_1801) -> cyemi_756/1, emi_2031/1, emi_2145/1
  emi_1804/1 -> cfblk13/Action
  emi_1804/2 -> emi_1802/Action
  emi_1805/1 -> emi_1804/1
  cyemi_752/1 -> cfblk3/1(emi_2026)
  cfblk3/1(emi_2027) -> cyemi_749/1
  emi_2030/1 -> cfblk3/Action
  emi_2030/2 -> emi_2028/Action
  emi_2031/1 -> emi_2030/1
  cyemi_750/1 -> cfblk12/1(emi_2140)
  cfblk12/1(emi_2141) -> emi_1805/1, emi_922/1, cyemi_755/1
  emi_2144/1 -> cfblk12/Action
  emi_2144/2 -> emi_2142/Action
  emi_2145/1 -> emi_2144/1

== system sampleModel7293_pp_1_1_mu/cfblk191 ==
  cfblk1 : Inport
  cfblk8 : Inport  Port=2
  Action Port : ActionPort  ActionType=else
  cfblk10 : Delay
  cfblk3 : DiscreteFir
  cfblk4 : simulink/Continuous/PID Controller (2DOF)  Controller=PID  TimeDomain=Discrete-time  SampleTime=-1  IntegratorMethod=Forward Euler  FilterMethod=Forward Euler  Form=Parallel  UseFilter=on  ControllerParametersSource=internal  P=1  I=1  D=0  N=100  b=1  c=1  InitialConditionSource=internal  InitialConditionForIntegrator=0  InitialConditionForFilter=0  ExternalReset=none  LimitOutput=off  UpperSaturationLimit=inf  LowerSaturationLimit=-inf  LinearizeAsGain=off  AntiWindupMode=none  Kb=1  TrackingMode=off  Kt=1  PParamMin=[]  PParamMax=[]  IParamMin=[]  IParamMax=[]  DParamMin=[]  DParamMax=[]  NParamMin=[]  NParamMax=[]  bParamMin=[]  bParamMax=[]  cParamMin=[]  cParamMax=[]  KbParamMin=[]  KbParamMax=[]  KtParamMin=[]  KtParamMax=[]  POutMin=[]  POutMax=[]  IOutMin=[]  IOutMax=[]  DOutMin=[]  DOutMax=[]  NOutMin=[]  NOutMax=[]  bOutMin=[]  bOutMax=[]  cOutMin=[]  cOutMax=[]  KbOutMin=[]  KbOutMax=[]  KtOutMin=[]  KtOutMax=[]  IntegratorOutMin=[]  IntegratorOutMax=[]  FilterOutMin=[]  FilterOutMax=[]  SumOutMin=[]  SumOutMax=[]  Sum1OutMin=[]  Sum1OutMax=[]  Sum2OutMin=[]  Sum2OutMax=[]  Sum3OutMin=[]  Sum3OutMax=[]  SumI1OutMin=[]  SumI1OutMax=[]  SumI2OutMin=[]  SumI2OutMax=[]  SumI3OutMin=[]  SumI3OutMax=[]  SumDOutMin=[]  SumDOutMax=[]  SaturationOutMin=[]  SaturationOutMax=[]  IntegratorContinuousStateAttributes=''  IntegratorStateMustResolveToSignalObject=off  IntegratorRTWStateStorageClass=Auto  FilterContinuousStateAttributes=''  FilterStateMustResolveToSignalObject=off  FilterRTWStateStorageClass=Auto  DifferentiatorICPrevScaledInput=0  DifferentiatorOutMin=[]  DifferentiatorOutMax=[]  FilterDiffOutCoefMin=[]  FilterDiffOutCoefMax=[]  SumDenOutMin=[]  SumDenOutMax=[]  SumNumOutMin=[]  SumNumOutMax=[]  ReciprocalOutMin=[]  ReciprocalOutMax=[]  DivideOutMin=[]  DivideOutMax=[]  TunerSelectOption=Transfer Function Based (PID Tuner App)
  cfblk5 : Subsystem  TreatAsAtomicUnit=on
  cfblk6 : Delay  DelayLengthSource=Input port
      settings: InputPortMap=u0,p1
  cfblk7 : DiscreteStateSpace  SampleTime=-1
  cfblk9 : Delay
  cyemi_{772..780} (9 alike) : DataTypeConversion  OutDataTypeStr=double
  emi_1218 : Subsystem  TreatAsAtomicUnit=on
  emi_1220 : If  IfExpression=0 <= u1
  emi_1221 : DataTypeConversion  OutDataTypeStr=double
  cfblk2 : Outport
  wires:
  cfblk8/1 -> cfblk2/1
  cfblk6/1 -> cyemi_773/1, cyemi_780/1, emi_1221/1
  cyemi_772/1 -> cfblk10/1
  cfblk3/1 -> cyemi_772/1
  cyemi_773/1 -> cfblk3/1
  cyemi_774/1 -> cfblk4/1
  cfblk7/1 -> cyemi_774/1
  cyemi_775/1 -> cfblk4/2
  cfblk9/1 -> cyemi_775/1
  cfblk1/1 -> cyemi_776/1
  cyemi_777/1 -> cfblk6/1
  cfblk4/1 -> cyemi_777/1
  cyemi_778/1 -> cfblk6/2
  cfblk10/1 -> cyemi_778/1
  cyemi_779/1 -> cfblk7/1
  cyemi_780/1 -> cfblk9/1
  cyemi_776/1 -> cfblk5/1(emi_1216)
  cfblk5/1(emi_1217) -> cyemi_779/1
  emi_1220/1 -> cfblk5/Action
  emi_1220/2 -> emi_1218/Action
  emi_1221/1 -> emi_1220/1

== system sampleModel7293_pp_1_1_mu/cfblk192 ==
  cfblk1 : Inport
  cfblk9 : Inport  Port=2
  cfblk10 : Inport  Port=3
  Action Port : ActionPort  ActionType=then
  cfblk3 : DiscreteTransferFcn
  cfblk4 : simulink/Discrete/Tapped Delay  vinit=0.0  samptime=-1  NumDelays=1  DelayOrder=Oldest  includeCurrent=off
  cfblk5 : DiscreteFir
  cfblk6 : Delay  DelayLengthSource=Input port
      settings: InputPortMap=u0,p1
  cfblk7 : simulink/Discrete/Difference  ICPrevInput=0.0  OutMin=[]  OutMax=[]  OutDataTypeStr=double  OutputDataTypeScalingMode=double  OutDataType=fixdt(1, 16)  OutScaling=2^-10  DoSatur=off
  cfblk8 : DiscreteTransferFcn
  cyemi_{784..790} (7 alike) : DataTypeConversion  OutDataTypeStr=double
  cfblk2 : Outport
  cfblk11 : Outport  Port=2
  wires:
  cfblk10/1 -> cfblk2/1
  cfblk5/1 -> cfblk11/1
  cyemi_784/1 -> cfblk3/1
  cfblk6/1 -> cyemi_784/1
  cyemi_785/1 -> cfblk4/1
  cfblk8/1 -> cyemi_785/1
  cyemi_786/1 -> cfblk5/1
  cfblk7/1 -> cyemi_786/1
  cyemi_787/1 -> cfblk6/1
  cfblk1/1 -> cyemi_787/1
  cyemi_788/1 -> cfblk6/2
  cfblk4/1 -> cyemi_788/1
  cyemi_789/1 -> cfblk7/1
  cfblk3/1 -> cyemi_789/1
  cyemi_790/1 -> cfblk8/1
  cfblk9/1 -> cyemi_790/1

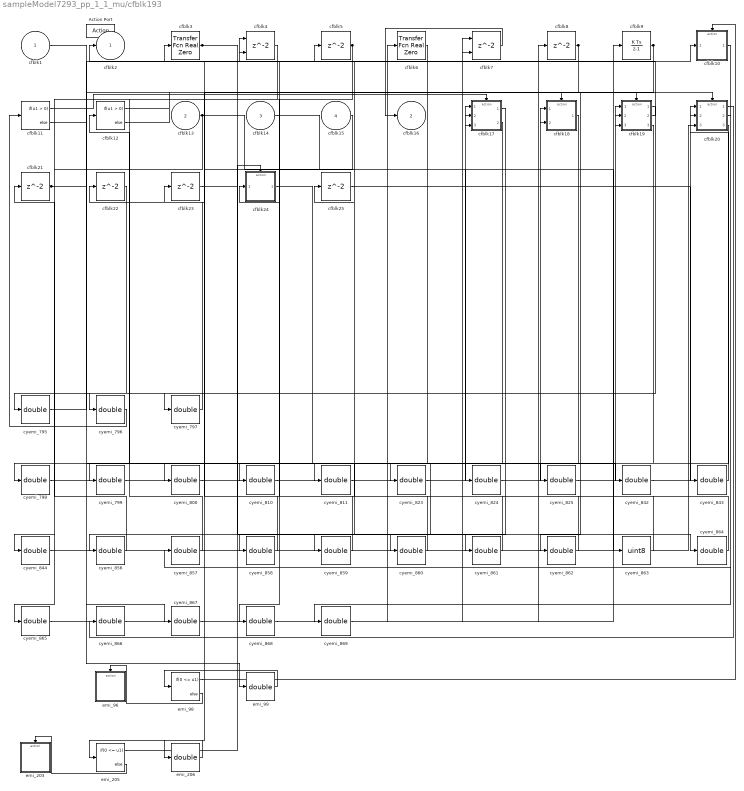
== system sampleModel7293_pp_1_1_mu/cfblk193 ==
  cfblk1 : Inport
  cfblk13 : Inport  Port=2
  cfblk14 : Inport  Port=3
  cfblk15 : Inport  Port=4
  Action Port : ActionPort  ActionType=else
  cfblk10 : Subsystem  TreatAsAtomicUnit=on
  cfblk11 : If  SampleTime=1
  cfblk12 : If  SampleTime=1
  cfblk17 : Subsystem  TreatAsAtomicUnit=on
  cfblk18 : Subsystem  TreatAsAtomicUnit=on
  cfblk19 : Subsystem  TreatAsAtomicUnit=on
  cfblk20 : Subsystem  TreatAsAtomicUnit=on
  cfblk{5,8,21..23,25} (6 alike) : Delay
  cfblk24 : Subsystem  TreatAsAtomicUnit=on
  cfblk3 : simulink/Discrete/Transfer Fcn Real Zero  ZeroZ=0.75  ICPrevInput=0.0  DoSatur=off
      settings: SourceProductName=Simulink  SourceProductBaseCode=SL
  cfblk4 : Delay  ShowEnablePort=on
      settings: InputPortMap=u0,e6
  cfblk6 : simulink/Discrete/Transfer Fcn Real Zero  ZeroZ=0.75  ICPrevInput=0.0  DoSatur=off
      settings: SourceProductName=Simulink  SourceProductBaseCode=SL
  cfblk7 : Delay  ShowEnablePort=on
      settings: InputPortMap=u0,e6
  cfblk9 : DiscreteIntegrator  SampleTime=-1  OutDataTypeStr=double  ICPrevOutput=DiscIntNeverNeededParam  ICPrevScaledInput=DiscIntNeverNeededParam
  cyemi_{795..800,810..811,823..825,842..844,856..862,864..869} (27 alike) : DataTypeConversion  OutDataTypeStr=double
  cyemi_863 : DataTypeConversion  OutDataTypeStr=uint8
  emi_203 : Subsystem  TreatAsAtomicUnit=on
  emi_205 : If  IfExpression=0 <= u1
  emi_206 : DataTypeConversion  OutDataTypeStr=double
  emi_96 : Subsystem  TreatAsAtomicUnit=on
  emi_98 : If  IfExpression=0 <= u1
  emi_99 : DataTypeConversion  OutDataTypeStr=double
  cfblk2 : Outport
  cfblk16 : Outport  Port=2
  wires:
  cfblk7/1 -> cfblk16/1
  cfblk5/1 -> cyemi_799/1, cyemi_868/1
  cfblk19/2(cfblk15) -> cfblk2/1
  cfblk8/1 -> cyemi_800/1, cyemi_823/1
  cfblk3/1 -> cyemi_811/1, cyemi_864/1
  cfblk13/1 -> cyemi_824/1, cyemi_844/1
  cfblk11/1 -> cfblk17/Action
  cfblk11/2 -> cfblk18/Action
  cfblk12/1 -> cfblk19/Action
  cfblk12/2 -> cfblk20/Action
  cfblk19/1(cfblk2) -> cyemi_795/1
  cyemi_796/1 -> cfblk11/1
  cfblk22/1 -> cyemi_796/1
  cyemi_797/1 -> cfblk12/1
  cfblk15/1 -> cyemi_797/1
  cyemi_798/1 -> cfblk17/1(cfblk1)
  cfblk4/1 -> cyemi_798/1
  cyemi_799/1 -> cfblk17/2(cfblk12)
  cyemi_800/1 -> cfblk17/3(cfblk13)
  cyemi_810/1 -> cfblk18/1(cfblk1)
  cfblk19/3(cfblk16) -> cyemi_810/1
  cyemi_811/1 -> cfblk18/2(cfblk11)
  cyemi_823/1 -> cfblk19/1(cfblk1)
  cyemi_824/1 -> cfblk19/2(cfblk13)
  cyemi_825/1 -> cfblk19/3(cfblk14)
  cyemi_842/1 -> cfblk20/1(cfblk1)
  cfblk21/1 -> cyemi_842/1, emi_99/1
  cyemi_843/1 -> cfblk20/2(cfblk13)
  cfblk25/1 -> cyemi_843/1
  cyemi_844/1 -> cfblk20/3(cfblk14)
  cyemi_856/1 -> cfblk21/1
  cfblk17/1(cfblk2) -> cyemi_856/1
  cyemi_857/1 -> cfblk22/1
  cfblk20/2(cfblk15) -> cyemi_857/1
  cyemi_858/1 -> cfblk23/1
  cfblk6/1 -> cyemi_858/1
  cfblk20/3(cfblk16) -> cyemi_859/1
  cyemi_860/1 -> cfblk25/1
  cfblk17/2(cfblk14) -> cyemi_860/1
  cyemi_861/1 -> cfblk3/1
  cfblk23/1 -> cyemi_861/1
  cyemi_862/1 -> cfblk4/1
  cfblk9/1 -> cyemi_862/1, emi_206/1
  cyemi_863/1 -> cfblk4/2
  cfblk14/1 -> cyemi_863/1
  cyemi_864/1 -> cfblk5/1
  cyemi_865/1 -> cfblk6/1
  cfblk18/1(cfblk2) -> cyemi_865/1
  cyemi_866/1 -> cfblk7/1
  cfblk20/1(cfblk2) -> cyemi_866/1
  cyemi_867/1 -> cfblk7/2
  cfblk1/1 -> cyemi_867/1
  cyemi_868/1 -> cfblk8/1
  cyemi_869/1 -> cfblk9/1
  cyemi_795/1 -> cfblk10/1(emi_94)
  cfblk10/1(emi_95) -> cyemi_869/1
  emi_98/1 -> cfblk10/Action
  emi_98/2 -> emi_96/Action
  emi_99/1 -> emi_98/1
  cyemi_859/1 -> cfblk24/1(emi_201)
  cfblk24/1(emi_202) -> cyemi_825/1
  emi_205/1 -> cfblk24/Action
  emi_205/2 -> emi_203/Action
  emi_206/1 -> emi_205/1

== system sampleModel7293_pp_1_1_mu/cfblk194 ==
  cfblk1 : Inport
  Action Port : ActionPort  ActionType=then
  cfblk3 : Delay
  cfblk4 : Subsystem  TreatAsAtomicUnit=on
  cfblk5 : Subsystem  TreatAsAtomicUnit=on
  cfblk6 : Subsystem  TreatAsAtomicUnit=on
  cfblk7 : Subsystem  TreatAsAtomicUnit=on
  cfblk8 : Subsystem  TreatAsAtomicUnit=on
  cyemi_{871..877} (7 alike) : DataTypeConversion  OutDataTypeStr=double
  emi_1730 : Subsystem  TreatAsAtomicUnit=on
  emi_{69,212,513,520,1732} (5 alike) : If  IfExpression=Inf <= u1
  emi_{70,213,514,521,1733} (5 alike) : DataTypeConversion  OutDataTypeStr=double
  emi_210 : Subsystem  TreatAsAtomicUnit=on
  emi_511 : Subsystem  TreatAsAtomicUnit=on
  emi_518 : Subsystem  TreatAsAtomicUnit=on
  emi_67 : Subsystem  TreatAsAtomicUnit=on
  cfblk2 : Outport
  wires:
  cyemi_871/1 -> cfblk3/1
  cfblk1/1 -> cyemi_873/1
  cfblk3/1 -> cyemi_874/1, emi_70/1, emi_1733/1
  cyemi_875/1 -> cfblk7/1(emi_64)
  cyemi_876/1 -> cfblk7/2(emi_65)
  cfblk7/1(emi_66) -> cyemi_872/1, emi_514/1
  emi_69/1 -> cfblk7/Action
  emi_69/2 -> emi_67/Action
  emi_70/1 -> emi_69/1
  cyemi_874/1 -> cfblk6/1(emi_208)
  cfblk6/1(emi_209) -> cyemi_877/1, cyemi_876/1
  emi_212/1 -> cfblk6/Action
  emi_212/2 -> emi_210/Action
  emi_213/1 -> emi_212/1
  cyemi_873/1 -> cfblk5/1(emi_509)
  cfblk5/1(emi_510) -> cyemi_875/1
  emi_513/1 -> cfblk5/Action
  emi_513/2 -> emi_511/Action
  emi_514/1 -> emi_513/1
  cyemi_872/1 -> cfblk4/1(emi_516)
  cfblk4/1(emi_517) -> cfblk2/1
  emi_520/1 -> cfblk4/Action
  emi_520/2 -> emi_518/Action
  emi_521/1 -> emi_520/1
  cyemi_877/1 -> cfblk8/1(emi_1728)
  cfblk8/1(emi_1729) -> emi_521/1, emi_213/1, cyemi_871/1
  emi_1732/1 -> cfblk8/Action
  emi_1732/2 -> emi_1730/Action
  emi_1733/1 -> emi_1732/1

== system sampleModel7293_pp_1_1_mu/cfblk195 ==
  cfblk1 : Inport
  cfblk7 : Inport  Port=2
  Action Port : ActionPort  ActionType=else
  cfblk10 : Delay
  cfblk11 : Subsystem  TreatAsAtomicUnit=on
  cfblk12 : Delay
  cfblk13 : Delay
  cfblk3 : Delay  ShowEnablePort=on
      settings: InputPortMap=u0,e6
  cfblk4 : Subsystem  TreatAsAtomicUnit=on
  cfblk5 : simulink/Discrete/Transfer Fcn Lead or Lag  PoleZ=0.95  ZeroZ=0.75  ICPrevOutput=0.0  ICPrevInput=0.0  DoSatur=off
      settings: SourceProductName=Simulink  SourceProductBaseCode=SL
  cfblk6 : If  SampleTime=1
  cfblk8 : Subsystem  TreatAsAtomicUnit=on
  cfblk9 : Subsystem  TreatAsAtomicUnit=on
  cyemi_{880..891,903..906} (16 alike) : DataTypeConversion  OutDataTypeStr=double
  emi_159 : Subsystem  TreatAsAtomicUnit=on
  emi_161 : If  IfExpression=0 <= u1
  emi_162 : DataTypeConversion  OutDataTypeStr=double
  emi_389 : Subsystem  TreatAsAtomicUnit=on
  emi_391 : If  IfExpression=0 <= u1
  emi_392 : DataTypeConversion  OutDataTypeStr=double
  cfblk2 : Outport
  wires:
  cfblk3/1 -> cyemi_883/1, cyemi_887/1
  cfblk5/1 -> cfblk2/1
  cfblk8/1(cfblk2) -> cyemi_880/1, cyemi_882/1, cyemi_886/1
  cfblk9/3(cfblk15) -> cyemi_885/1, cyemi_891/1
  cfblk6/1 -> cfblk8/Action
  cfblk6/2 -> cfblk9/Action
  cyemi_880/1 -> cfblk10/1
  cyemi_882/1 -> cfblk12/1
  cyemi_883/1 -> cfblk13/1
  cyemi_884/1 -> cfblk3/1
  cfblk7/1 -> cyemi_884/1
  cyemi_885/1 -> cfblk3/2
  cyemi_887/1 -> cfblk5/1
  cyemi_888/1 -> cfblk6/1
  cyemi_889/1 -> cfblk8/1(cfblk1)
  cfblk9/1(cfblk2) -> cyemi_889/1
  cyemi_890/1 -> cfblk8/2(cfblk11)
  cfblk9/2(cfblk14) -> cyemi_890/1
  cyemi_891/1 -> cfblk8/3(cfblk12)
  cyemi_903/1 -> cfblk9/1(cfblk1)
  cfblk10/1 -> cyemi_903/1
  cyemi_904/1 -> cfblk9/2(cfblk11)
  cfblk1/1 -> cyemi_904/1
  cyemi_905/1 -> cfblk9/3(cfblk12)
  cfblk13/1 -> cyemi_905/1, emi_162/1, emi_392/1
  cyemi_906/1 -> cfblk9/4(cfblk13)
  cfblk12/1 -> cyemi_906/1
  cyemi_881/1 -> cfblk11/1(emi_157)
  cfblk11/1(emi_158) -> cyemi_888/1
  emi_161/1 -> cfblk11/Action
  emi_161/2 -> emi_159/Action
  emi_162/1 -> emi_161/1
  cyemi_886/1 -> cfblk4/1(emi_387)
  cfblk4/1(emi_388) -> cyemi_881/1
  emi_391/1 -> cfblk4/Action
  emi_391/2 -> emi_389/Action
  emi_392/1 -> emi_391/1

== system sampleModel7293_pp_1_1_mu/cfblk196 ==
  cfblk1 : Inport
  cfblk9 : Inport  Port=2
  cfblk10 : Inport  Port=3
  Action Port : ActionPort  ActionType=then
  cfblk11 : Subsystem  TreatAsAtomicUnit=on
  cfblk12 : Subsystem  TreatAsAtomicUnit=on
  cfblk13 : Delay
  cfblk14 : Delay
  cfblk3 : Subsystem  TreatAsAtomicUnit=on
  cfblk4 : Subsystem  TreatAsAtomicUnit=on
  cfblk5 : Delay  ShowEnablePort=on
      settings: InputPortMap=u0,e6
  cfblk6 : DiscreteStateSpace  SampleTime=-1
  cfblk7 : Subsystem  TreatAsAtomicUnit=on
  cfblk8 : If  SampleTime=1
  cyemi_{919..921,929,940..948} (13 alike) : DataTypeConversion  OutDataTypeStr=double
  emi_1659 : Subsystem  TreatAsAtomicUnit=on
  emi_1661 : If  IfExpression=Inf <= u1
  emi_1662 : DataTypeConversion  OutDataTypeStr=double
  emi_231 : Subsystem  TreatAsAtomicUnit=on
  emi_233 : If  IfExpression=Inf <= u1
  emi_234 : DataTypeConversion  OutDataTypeStr=double
  emi_310 : Subsystem  TreatAsAtomicUnit=on
  emi_312 : If  IfExpression=Inf <= u1
  emi_313 : DataTypeConversion  OutDataTypeStr=double
  cfblk2 : Outport
  wires:
  cfblk12/1(cfblk2) -> cfblk2/1
  cfblk8/1 -> cfblk11/Action
  cfblk8/2 -> cfblk12/Action
  cyemi_919/1 -> cfblk11/1(cfblk1)
  cfblk14/1 -> cyemi_919/1
  cyemi_920/1 -> cfblk11/2(cfblk10)
  cfblk1/1 -> cyemi_920/1, cyemi_921/1
  cyemi_921/1 -> cfblk11/3(cfblk11)
  cyemi_929/1 -> cfblk12/1(cfblk1)
  cyemi_940/1 -> cfblk13/1
  cfblk5/1 -> cyemi_940/1
  cyemi_941/1 -> cfblk14/1
  cfblk10/1 -> cyemi_942/1
  cyemi_944/1 -> cfblk5/1
  cfblk9/1 -> cyemi_944/1
  cyemi_945/1 -> cfblk5/2
  cfblk11/1(cfblk2) -> cyemi_945/1
  cyemi_946/1 -> cfblk6/1
  cfblk12/2(cfblk12) -> cyemi_946/1
  cfblk6/1 -> cyemi_947/1, emi_234/1
  cyemi_948/1 -> cfblk8/1
  cfblk13/1 -> cyemi_948/1, emi_1662/1
  cyemi_942/1 -> cfblk3/1(emi_229)
  cfblk3/1(emi_230) -> cyemi_943/1
  emi_233/1 -> cfblk3/Action
  emi_233/2 -> emi_231/Action
  emi_234/1 -> emi_233/1
  cyemi_943/1 -> cfblk4/1(emi_308)
  cfblk4/1(emi_309) -> cyemi_929/1
  emi_312/1 -> cfblk4/Action
  emi_312/2 -> emi_310/Action
  emi_313/1 -> emi_312/1
  cyemi_947/1 -> cfblk7/1(emi_1657)
  cfblk7/1(emi_1658) -> emi_313/1, cyemi_941/1
  emi_1661/1 -> cfblk7/Action
  emi_1661/2 -> emi_1659/Action
  emi_1662/1 -> emi_1661/1
